simulink model "VendingMachine"  (R2020b)
settings: Solver=VariableStepAuto  StartTime=0.0  StopTime=100  RelTol=1e-3
libraries: simulink x1
settings Model: Creator=Shree  LastModifiedBy=Shree

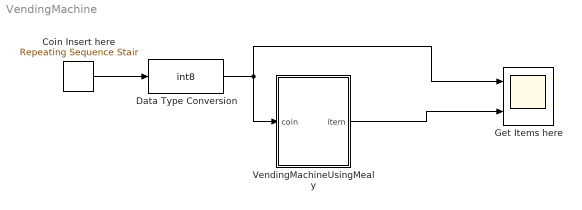
== system VendingMachine ==
  Coin Insert here : simulink/Sources/Repeating Sequence Stair  OutValues=[0 0 1 1 2 2 2 1 1 1 0 0 2]';  tsamp=-1  OutMin=[]  OutMax=[]  OutDataTypeStr=double  OutputDataTypeScalingMode=double  OutDataType=fixdt(0,8)  ConRadixGroup=Best Precision: Vector-wise  OutScaling=2^-12
  Data Type Conversion : DataTypeConversion  OutDataTypeStr=int8
  Get Items here : Scope  NumInputPorts=2
  VendingMachineUsingMealy : Stateflow chart  TreatAsAtomicUnit=on
  wires:
  Coin Insert here/1 -> Data Type Conversion/1
  Data Type Conversion/1 -> VendingMachineUsingMealy/1(coin), Get Items here/1
  VendingMachineUsingMealy/1(item) -> Get Items here/2

== stateflow chart VendingMachine/VendingMachineUsingMealy ==
  state Coin_0
  state Coin_2
  state Coin_1
  (default) -> Coin_0
  Coin_2 -> Coin_0 [order 1] : [coin==1]{item=1}
  Coin_0 -> Coin_1 [order 1] : [coin==1]{item=0}
  Coin_0 -> Coin_2 [order 2] : [coin==2]{item=0}
  Coin_1 -> Coin_0 [order 2] : [coin==2]{item=1}
  Coin_1 -> Coin_2 [order 1] : [coin==1]{item=0}
  Coin_2 -> Coin_1 [order 2] : [coin==2]{item=1}
  data: coin input; item output
